simulink model "Main"  (R2022a)
settings: Solver=VariableStepAuto  StartTime=0.0  StopTime=30  RelTol=1e-3
values from neighbouring files (symbols this model uses):
  A_eq = double(A_eq)    [source_export.m]
  b = 7.66e-5    (= 7.66e-05)    [source_export.m]
  B_eq = double(B_eq)    [source_export.m]
  C = [1 0 0 0 0 0 0 0 0 0 0 0 ... (first row only)    [source_export.m]
  C_eq = C_final([1 2 3 6], 1:12)    [source_export.m]
  C_simulink = eye(12)    [source_export.m]
  Condition_0 = transpose([0 0 0 0 0 0 0 0 0 0 0 0])    [source_export.m]
  Condition_1 = transpose([0.2 0.2 0.2 0.2 0.2 0.2 0.2 0.2 0.2 0.2 0.2 0.2])    [source_export.m]
  D = zeros(4,4)    [source_export.m]
  d = 5.63e-6    (= 5.63e-06)    [source_export.m]
  D_Simulink = zeros(12,4)    [source_export.m]
  F = [      -20,   -20,   -20,   -21,   -21,   15,   -21.5, -21.5 ... (first row only)    [source_export.m]
  g = 9.81    [source_export.m]
  inv_G0 = inv_G_0( : , [1 , 2 ,3 ,6])    [source_export.m]
  inv_G0_LQR = inv_G_0_LQR( : , [1 , 2 ,3 ,6])    [source_export.m]
  Ixx = 8.5532e-3    (= 0.0085532)    [source_export.m]
  Iyy = 8.5532e-3    (= 0.0085532)    [source_export.m]
  Izz = 1.476e-2    (= 0.01476)    [source_export.m]
  K_d_LQR = K_LQR(:,1:12)    [source_export.m]
  K_q_LQR = K_LQR(:,12+1:12+4)    [source_export.m]
  Kfeedback = place(A_eq,B_eq,Poles)    [source_export.m]
  L = place(A_eq.',C_eq.',poles_obsv).'    [source_export.m]
  l = 0.22    [source_export.m]
  L_RO = 100*[1 2 1 14 ... (first row only)    [source_export.m]
  m = 1    [source_export.m]
  Q_1 = inv_mat2(:,1:q)    [source_export.m]
  Q_2 = inv_mat2(:,q+1:n)    [source_export.m]
  T_O = lyap(-F,A_eq,-L_RO*C)    [source_export.m]
undefined symbols (not defined in the file or in its folder): Discrete, K_LQR1, Time
libraries: slpidlib x8, simulink x6, ctrlSharedLib x1, sim3dlib x1, uavsim3dlib x1
(part 2 of 2)

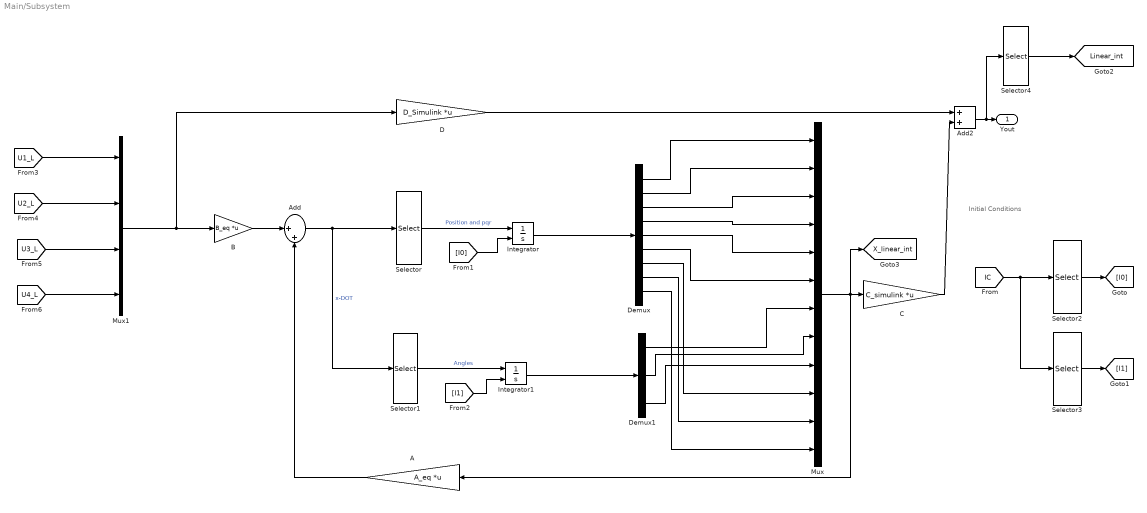
== system Main/Subsystem ==
  note: Initial Conditions
  A : Gain  Gain=A_eq  Multiplication=Matrix(K*u)
  Add : Sum  Inputs=|++
  Add2 : Sum
  B : Gain  Gain=B_eq  Multiplication=Matrix(K*u)
  C : Gain  Gain=C_simulink  Multiplication=Matrix(K*u)
  D : Gain  Gain=D_Simulink  Multiplication=Matrix(K*u)
  Demux : Demux  Outputs=9
  Demux1 : Demux  Outputs=3
  Integrator : Integrator  InitialConditionSource=external
  Integrator1 : Integrator  InitialConditionSource=external  WrapState=on
  Mux : Mux  Inputs=12
  Mux1 : Mux
  Selector : Selector  InputPortWidth=12  IndexOptions=Index vector (dialog)  Indices=[1 2 3 4 5 6 10 11 12]  OutputSizes=1
  Selector1 : Selector  InputPortWidth=12  IndexOptions=Index vector (dialog)  Indices=[7 8 9]  OutputSizes=1
  Selector2 : Selector  InputPortWidth=12  IndexOptions=Index vector (dialog)  Indices=[1 2 3 4 5 6 10 11 12]  OutputSizes=1
  Selector3 : Selector  InputPortWidth=12  IndexOptions=Index vector (dialog)  Indices=[7 8 9]  OutputSizes=1
  Selector4 : Selector  InputPortWidth=12  IndexOptions=Index vector (dialog)  Indices=[1 3 5 7 8 9]  OutputSizes=1
  Yout : Outport
  tag scope: Linear_int=global, X_linear_int=global
  wires:
  B/1 -> Add/1
  A/1 -> Add/2
  Add/1 -> Selector1/1, Selector/1  "x-DOT"
  Selector/1 -> Integrator/1  "Position and pqr"
  Selector1/1 -> Integrator1/1  "Angles"
  [IC] -> Selector3/1, Selector2/1
  Selector3/1 -> [I1]
  Selector2/1 -> [I0]
  [I1] -> Integrator1/2
  [I0] -> Integrator/2
  Integrator1/1 -> Demux1/1
  Integrator/1 -> Demux/1
  Demux/1 -> Mux/1
  Demux/2 -> Mux/2
  Demux/3 -> Mux/3
  Demux/4 -> Mux/4
  Demux/5 -> Mux/5
  Demux/6 -> Mux/6
  Demux1/1 -> Mux/7
  Demux1/2 -> Mux/8
  Demux1/3 -> Mux/9
  Demux/7 -> Mux/10
  Demux/8 -> Mux/11
  Demux/9 -> Mux/12
  D/1 -> Add2/1
  C/1 -> Add2/2
  Mux1/1 -> D/1, B/1
  [U2_L] -> Mux1/2
  [U3_L] -> Mux1/3
  [U4_L] -> Mux1/4
  Add2/1 -> Selector4/1, Yout/1
  Mux/1 -> [X_linear_int], A/1, C/1
  [U1_L] -> Mux1/1
  Selector4/1 -> [Linear_int]

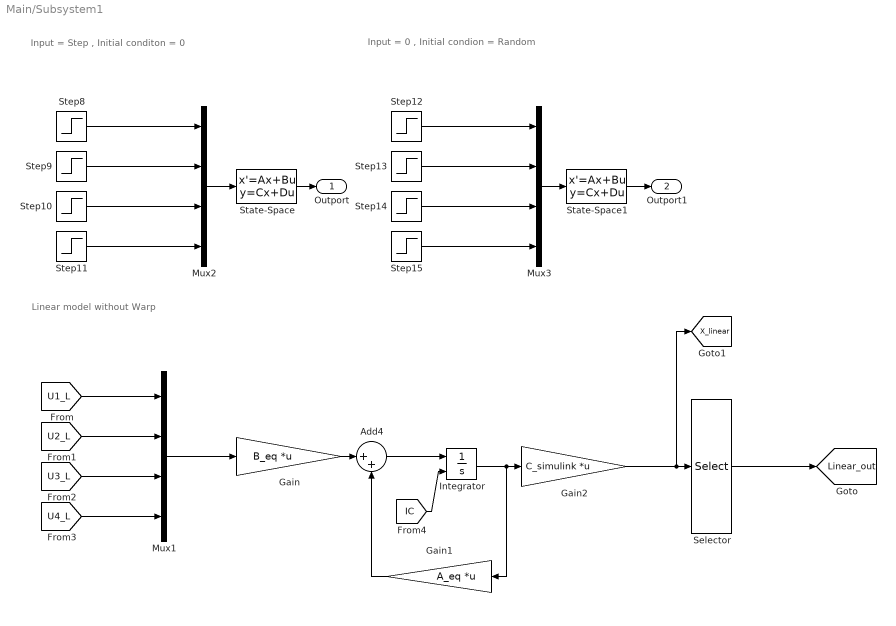
== system Main/Subsystem1 ==
  note: Linear model without Warp
  note: Input = Step , Initial conditon = 0
  note: Input = 0 , Initial condion = Random
  Add4 : Sum  Inputs=|++
  Gain : Gain  Gain=B_eq  Multiplication=Matrix(K*u)
  Gain1 : Gain  Gain=A_eq  Multiplication=Matrix(K*u)
  Gain2 : Gain  Gain=C_simulink  Multiplication=Matrix(K*u)
  Integrator : Integrator  InitialConditionSource=external
  Mux1 : Mux
  Mux2 : Mux
  Mux3 : Mux
  Selector : Selector  InputPortWidth=12  IndexOptions=Index vector (dialog)  Indices=[1 3 5 7 8 9]  OutputSizes=1
  State-Space : StateSpace  A=A_eq  B=B_eq  C=C  D=D  InitialCondition=Condition_0
  State-Space1 : StateSpace  A=A_eq  B=B_eq  C=C  D=D  InitialCondition=Condition_1
  Step{8..11} (4 alike) : Step  Time=0  SampleTime=0
  Step{12..15} (4 alike) : Step  Time=0  After=0  SampleTime=0
  Outport : Outport
  Outport1 : Outport  Port=2
  tag scope: Linear_out=global, X_linear=global
  wires:
  State-Space1/1 -> Outport1/1
  Step15/1 -> Mux3/4
  Step11/1 -> Mux2/4
  Step9/1 -> Mux2/2
  Mux3/1 -> State-Space1/1
  Step10/1 -> Mux2/3
  State-Space/1 -> Outport/1
  Step13/1 -> Mux3/2
  Mux2/1 -> State-Space/1
  Step14/1 -> Mux3/3
  [U2_L] -> Mux1/2
  [U3_L] -> Mux1/3
  [U4_L] -> Mux1/4
  Step12/1 -> Mux3/1
  [U1_L] -> Mux1/1
  Selector/1 -> [Linear_out]
  [IC] -> Integrator/2
  Integrator/1 -> Gain1/1, Gain2/1
  Gain1/1 -> Add4/2
  Mux1/1 -> Gain/1
  Gain/1 -> Add4/1
  Gain2/1 -> [X_linear], Selector/1
  Add4/1 -> Integrator/1
  Step8/1 -> Mux2/1

== system Main/Subsystem2 ==
  In1 : Inport
  Demux8 : Demux
  tag scope: i1=global, i2=global, i3=global, i4=global
  wires:
  In1/1 -> Demux8/1
  Demux8/1 -> [i1]
  Demux8/2 -> [i2]
  Demux8/3 -> [i3]
  Demux8/4 -> [i4]

== system Main/Subsystem3 ==
  Translation : Inport
  Rotation : Inport  Port=2
  Simulation 3D Scene Configuration : sim3dlib/Simulation 3D Scene Configuration  Priority=0  ProjectFormat=Default Scenes  SceneDesc=US city block  ProjectName=C:\Program Files\MATLAB\R2022b\toolbox\shared\sim3d_projects\automotive_project\UE4\WindowsNoEditor\VehicleSimulation.exe  ScenePath=/Game/Maps/USCityBlock  EnableOpenDRIVE=off  vehTagList={'Scene Origin';'SimulinkVehicle1'}  vehTag=SimulinkVehicle1  OpVisEn=off  Ts=1/60  EnableWindow=on  EnableRemoteAccess=off  EnableWeather=on  SunAltitude=90.0  SunAzimuth=147.600  clouds=26.0  wind=1  fog=14.0  rain=4.0  sensorTag=MainCamera1  sensorId=1  sensorName=MainCamera1  mountLoc=Origin  offsetFlag=off  tmountOffset=[0, 0, 0]  rmountOffset=[0, 0, 0]  HorizontalResolution=1280  VerticalResolution=720  HorizontalFOV=60  mountPoint=[0 0 0]  mountOrientation=[0 0 0]  aMode=4  ID=1  GeoTrigger=Inactive
  Simulation 3D UAV Vehicle : uavsim3dlib/Simulation 3D UAV Vehicle  Priority=-1  Mesh=Quadrotor  MeshPath=/MathWorksUAVContent/UAVs/HexaRotorUAV/HexaRotor.HexaRotor  Color=Black  ActorName=SimulinkVehicle1  InitialTranslation=[0 0 1]  InitialRotation=[0 0 0]  SampleTime=-1  ActorType=SimulinkVehicle  ID=1  aMode=4  ActorTag=SimulinkVehicle1
  wires:
  Rotation/1 -> Simulation 3D UAV Vehicle/2
  Translation/1 -> Simulation 3D UAV Vehicle/1

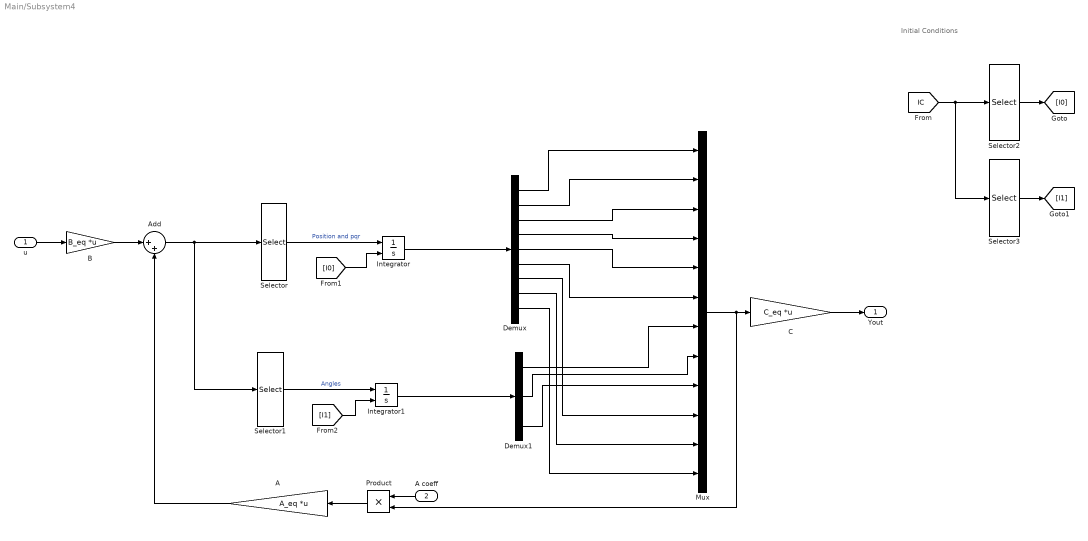
== system Main/Subsystem4 ==
  note: Initial Conditions
  u : Inport
  A coeff : Inport  Port=2
  A : Gain  Gain=A_eq  Multiplication=Matrix(K*u)
  Add : Sum  Inputs=|++
  B : Gain  Gain=B_eq  Multiplication=Matrix(K*u)
  C : Gain  Gain=C_eq  Multiplication=Matrix(K*u)
  Demux : Demux  Outputs=9
  Demux1 : Demux  Outputs=3
  Integrator : Integrator  InitialConditionSource=external
  Integrator1 : Integrator  InitialConditionSource=external  WrapState=on
  Mux : Mux  Inputs=12
  Product : Product
  Selector : Selector  InputPortWidth=12  IndexOptions=Index vector (dialog)  Indices=[1 2 3 4 5 6 10 11 12]  OutputSizes=1
  Selector1 : Selector  InputPortWidth=12  IndexOptions=Index vector (dialog)  Indices=[7 8 9]  OutputSizes=1
  Selector2 : Selector  InputPortWidth=12  IndexOptions=Index vector (dialog)  Indices=[1 2 3 4 5 6 10 11 12]  OutputSizes=1
  Selector3 : Selector  InputPortWidth=12  IndexOptions=Index vector (dialog)  Indices=[7 8 9]  OutputSizes=1
  Yout : Outport
  wires:
  B/1 -> Add/1
  A/1 -> Add/2
  Add/1 -> Selector1/1, Selector/1
  Selector/1 -> Integrator/1  "Position and pqr"
  Selector1/1 -> Integrator1/1  "Angles"
  [IC] -> Selector3/1, Selector2/1
  Selector3/1 -> [I1]
  Selector2/1 -> [I0]
  [I1] -> Integrator1/2
  [I0] -> Integrator/2
  Integrator1/1 -> Demux1/1
  Integrator/1 -> Demux/1
  Demux/1 -> Mux/1
  Demux/2 -> Mux/2
  Demux/3 -> Mux/3
  Demux/4 -> Mux/4
  Demux/5 -> Mux/5
  Demux/6 -> Mux/6
  Demux1/1 -> Mux/7
  Demux1/2 -> Mux/8
  Demux1/3 -> Mux/9
  Demux/7 -> Mux/10
  Demux/8 -> Mux/11
  Demux/9 -> Mux/12
  Mux/1 -> Product/2, C/1
  C/1 -> Yout/1
  u/1 -> B/1
  Product/1 -> A/1
  A coeff/1 -> Product/1

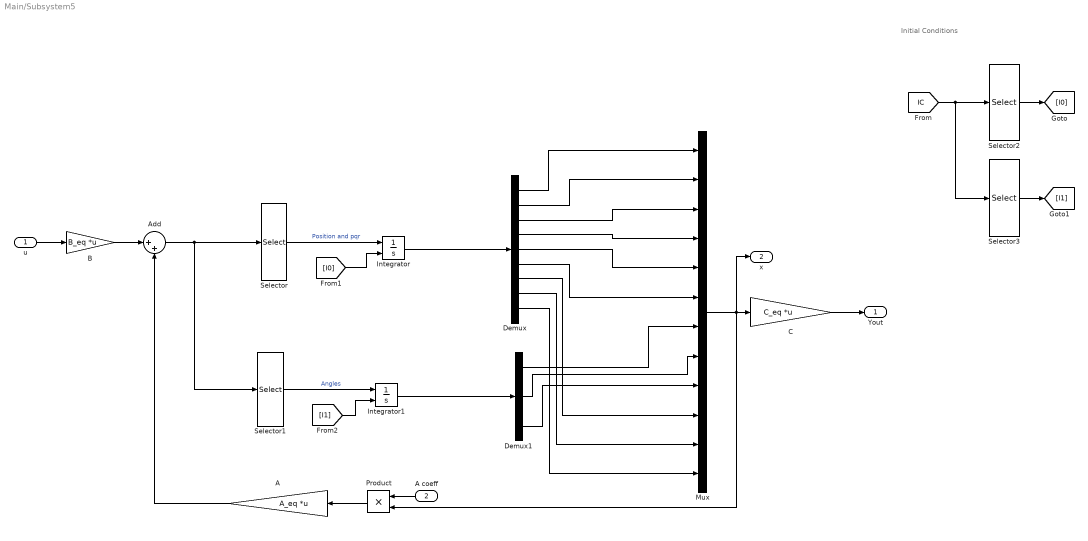
== system Main/Subsystem5 ==
  note: Initial Conditions
  u : Inport
  A coeff : Inport  Port=2
  A : Gain  Gain=A_eq  Multiplication=Matrix(K*u)
  Add : Sum  Inputs=|++
  B : Gain  Gain=B_eq  Multiplication=Matrix(K*u)
  C : Gain  Gain=C_eq  Multiplication=Matrix(K*u)
  Demux : Demux  Outputs=9
  Demux1 : Demux  Outputs=3
  Integrator : Integrator  InitialConditionSource=external
  Integrator1 : Integrator  InitialConditionSource=external  WrapState=on
  Mux : Mux  Inputs=12
  Product : Product
  Selector : Selector  InputPortWidth=12  IndexOptions=Index vector (dialog)  Indices=[1 2 3 4 5 6 10 11 12]  OutputSizes=1
  Selector1 : Selector  InputPortWidth=12  IndexOptions=Index vector (dialog)  Indices=[7 8 9]  OutputSizes=1
  Selector2 : Selector  InputPortWidth=12  IndexOptions=Index vector (dialog)  Indices=[1 2 3 4 5 6 10 11 12]  OutputSizes=1
  Selector3 : Selector  InputPortWidth=12  IndexOptions=Index vector (dialog)  Indices=[7 8 9]  OutputSizes=1
  Yout : Outport
  x : Outport  Port=2
  wires:
  B/1 -> Add/1
  A/1 -> Add/2
  Add/1 -> Selector1/1, Selector/1
  Selector/1 -> Integrator/1  "Position and pqr"
  Selector1/1 -> Integrator1/1  "Angles"
  [IC] -> Selector3/1, Selector2/1
  Selector3/1 -> [I1]
  Selector2/1 -> [I0]
  [I1] -> Integrator1/2
  [I0] -> Integrator/2
  Integrator1/1 -> Demux1/1
  Integrator/1 -> Demux/1
  Demux/1 -> Mux/1
  Demux/2 -> Mux/2
  Demux/3 -> Mux/3
  Demux/4 -> Mux/4
  Demux/5 -> Mux/5
  Demux/6 -> Mux/6
  Demux1/1 -> Mux/7
  Demux1/2 -> Mux/8
  Demux1/3 -> Mux/9
  Demux/7 -> Mux/10
  Demux/8 -> Mux/11
  Demux/9 -> Mux/12
  Mux/1 -> Product/2, x/1, C/1
  C/1 -> Yout/1
  u/1 -> B/1
  Product/1 -> A/1
  A coeff/1 -> Product/1

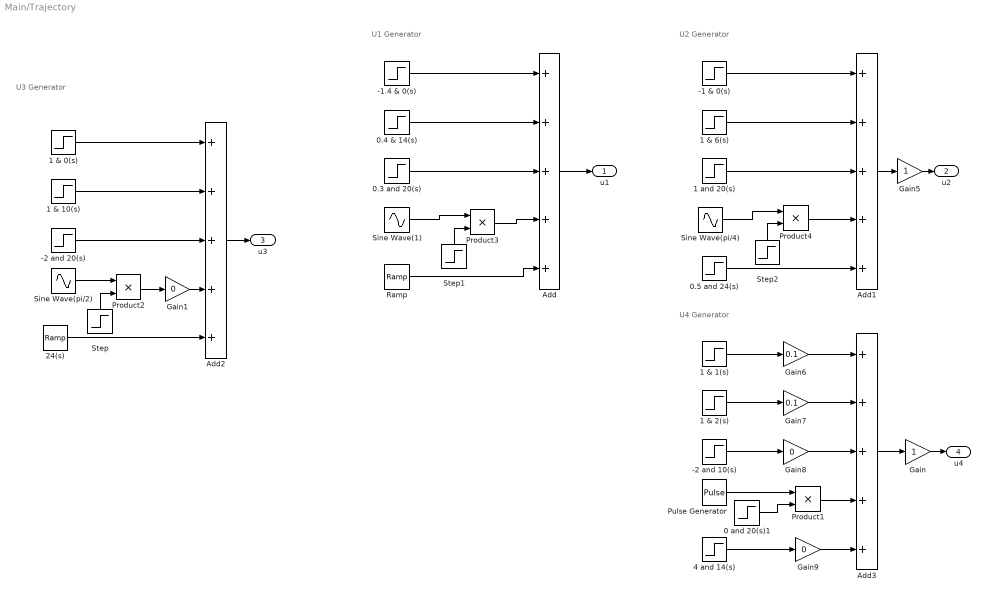
== system Main/Trajectory  ==
  note: U4 Generator
  note: U3 Generator
  note: U2 Generator
  note: U1 Generator
  -1 & 0(s) : Step  Time=0  After=-1  SampleTime=0
  -1.4 & 0(s) : Step  Time=0  After=-1.4  SampleTime=0
  -2 and 10(s) : Step  Time=10  After=-2  SampleTime=0
  -2 and 20(s) : Step  Time=20  After=-2  SampleTime=0
  0 and 20(s)1 : Step  Time=20  Before=1  After=0  SampleTime=0
  0.3 and 20(s) : Step  Time=20  After=0.3  SampleTime=0
  0.4 & 14(s) : Step  Time=14  After=0.4  SampleTime=0
  0.5 and 24(s) : Step  Time=24  After=0.5  SampleTime=0
  1 & 0(s) : Step  Time=0  After=2  SampleTime=0
  1 & 1(s) : Step  SampleTime=0
  1 & 10(s) : Step  Time=10  After=2  SampleTime=0
  1 & 2(s) : Step  Time=2  After=-1  SampleTime=0
  1 & 6(s) : Step  Time=6  SampleTime=0
  1 and 20(s) : Step  Time=20  SampleTime=0
  24(s) : simulink/Sources/Ramp  slope=1  start=24  InitialOutput=0
  4 and 14(s) : Step  Time=12  After=4  SampleTime=0
  Add{,1..3} (4 alike) : Sum  Inputs=+++++
  Gain : Gain
  Gain1 : Gain  Gain=0
  Gain5 : Gain
  Gain6 : Gain  Gain=0.1
  Gain7 : Gain  Gain=0.1
  Gain8 : Gain  Gain=0
  Gain9 : Gain  Gain=0
  Product{1..4} (4 alike) : Product
  Pulse Generator : DiscretePulseGenerator  PulseType=Time based  Period=5  PulseWidth=30  PhaseDelay=5
  Ramp : simulink/Sources/Ramp  slope=2  start=0  InitialOutput=0
  Sine Wave(1) : Sin  Amplitude=0.4  SampleTime=0
  Sine Wave(pi/2) : Sin  Amplitude=0.4  Frequency=pi/2  SampleTime=0
  Sine Wave(pi/4) : Sin  Frequency=pi/4  SampleTime=0
  Step : Step  Time=6  SampleTime=0
  Step1 : Step  Time=8  SampleTime=0
  Step2 : Step  Time=11  SampleTime=0
  u1 : Outport
  u2 : Outport  Port=2
  u3 : Outport  Port=3
  u4 : Outport  Port=4
  wires:
  Add/1 -> u1/1
  -1.4 & 0(s)/1 -> Add/1
  0.3 and 20(s)/1 -> Add/3
  0.4 & 14(s)/1 -> Add/2
  Ramp/1 -> Add/5
  0.5 and 24(s)/1 -> Add1/5
  1 & 6(s)/1 -> Add1/2
  -1 & 0(s)/1 -> Add1/1
  1 and 20(s)/1 -> Add1/3
  Add2/1 -> u3/1
  -2 and 20(s)/1 -> Add2/3
  24(s)/1 -> Add2/5
  Sine Wave(pi/2)/1 -> Product2/1
  1 & 10(s)/1 -> Add2/2
  1 & 0(s)/1 -> Add2/1
  Product2/1 -> Gain1/1
  Add3/1 -> Gain/1
  4 and 14(s)/1 -> Gain9/1
  1 & 1(s)/1 -> Gain6/1
  -2 and 10(s)/1 -> Gain8/1
  1 & 2(s)/1 -> Gain7/1
  Gain/1 -> u4/1
  Gain1/1 -> Add2/4
  Product4/1 -> Add1/4
  Add1/1 -> Gain5/1
  Gain5/1 -> u2/1
  Gain6/1 -> Add3/1
  Gain7/1 -> Add3/2
  Gain8/1 -> Add3/3
  Gain9/1 -> Add3/5
  Product1/1 -> Add3/4
  Pulse Generator/1 -> Product1/1
  0 and 20(s)1/1 -> Product1/2
  Step/1 -> Product2/2
  Sine Wave(1)/1 -> Product3/1
  Step1/1 -> Product3/2
  Product3/1 -> Add/4
  Sine Wave(pi/4)/1 -> Product4/1
  Step2/1 -> Product4/2

== system Main/pqr ==
  Integrator1 : Integrator  InitialConditionSource=external
  Integrator2 : Integrator  InitialConditionSource=external
  Integrator3 : Integrator  InitialConditionSource=external
  tag scope: p=global, q=global, r=global
  wires:
  [q0] -> Integrator2/2
  [q_dot] -> Integrator2/1
  Integrator2/1 -> [q]
  Integrator1/1 -> [p]
  [p_dot] -> Integrator1/1
  [p0] -> Integrator1/2
  [r_dot] -> Integrator3/1
  [r0] -> Integrator3/2
  Integrator3/1 -> [r]

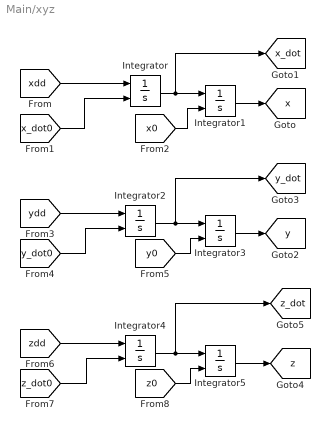
== system Main/xyz ==
  Integrator{,1..5} (6 alike) : Integrator  InitialConditionSource=external
  tag scope: x=global, x_dot=global, y=global, y_dot=global, z=global, z_dot=global
  wires:
  Integrator3/1 -> [y]
  [z0] -> Integrator5/2
  [x0] -> Integrator1/2
  Integrator2/1 -> [y_dot], Integrator3/1
  [y0] -> Integrator3/2
  Integrator/1 -> Integrator1/1, [x_dot]
  Integrator1/1 -> [x]
  Integrator4/1 -> [z_dot], Integrator5/1
  Integrator5/1 -> [z]
  [z_dot0] -> Integrator4/2
  [zdd] -> Integrator4/1
  [y_dot0] -> Integrator2/2
  [ydd] -> Integrator2/1
  [x_dot0] -> Integrator/2
  [xdd] -> Integrator/1

== system Main/Full order Observer/Dynamic Pre-compensator Observer ==
  x_hat_L : Inport
  y : Inport  Port=2
  u : Inport  Port=3
  Add : Sum  Inputs=+-
  Add3 : Sum  Inputs=--
  Integrator1 : Integrator
  Matrix Multiply1 : Product  Multiplication=Matrix(*)
  Matrix Multiply3 : Product  Multiplication=Matrix(*)
  Linear Sys input : Outport
  wires:
  u/1 -> Add/1
  y/1 -> Add/2
  Add/1 -> Integrator1/1
  Integrator1/1 -> Matrix Multiply1/2
  [Gain_Dynamic] -> Matrix Multiply1/1
  [Gain_Dyn_State] -> Matrix Multiply3/1
  x_hat_L/1 -> Matrix Multiply3/2
  Matrix Multiply1/1 -> Add3/1
  Matrix Multiply3/1 -> Add3/2
  Add3/1 -> Linear Sys input/1

== system Main/Full order Observer/Full Order Observer  ==
  y_L : Inport
  u_L - kx : Inport  Port=2
  Add2 : Sum  Inputs=+-
  Add3 : Sum  Inputs=+++
  Constant4 : Constant  Value=C_eq
  Constant5 : Constant  Value=A_eq
  Constant6 : Constant  Value=L
  Constant7 : Constant  Value=B_eq
  Integrator1 : Integrator  InitialConditionSource=external
  MatrixMultiply{4..7} (4 alike) : Product  Multiplication=Matrix(*)
  Scope : Scope
  x_hat_L : Outport
  wires:
  MatrixMultiply6/1 -> Add3/1, Scope/1  "L(y-Cx_hat)"
  Constant6/1 -> MatrixMultiply6/1
  MatrixMultiply4/1 -> Add2/2
  y_L/1 -> Add2/1
  Constant5/1 -> MatrixMultiply5/1
  Add2/1 -> MatrixMultiply6/2  "y - Cx_hat"
  u_L - kx/1 -> MatrixMultiply7/2
  Add3/1 -> Integrator1/1  "x_hat_dot"
  MatrixMultiply7/1 -> Add3/3  "Bu"
  MatrixMultiply5/1 -> Add3/2  "Ax_hat"
  Constant7/1 -> MatrixMultiply7/1
  Integrator1/1 -> x_hat_L/1, MatrixMultiply5/2, MatrixMultiply4/2
  Constant4/1 -> MatrixMultiply4/1

== system Main/Full order Observer/Full Order Observer Dynamic ==
  u_L - kx : Inport
  y_L : Inport  Port=2
  Add2 : Sum  Inputs=+-
  Add3 : Sum  Inputs=+++
  Constant4 : Constant  Value=C_eq
  Constant5 : Constant  Value=A_eq
  Constant6 : Constant  Value=L
  Constant7 : Constant  Value=B_eq
  Integrator1 : Integrator  InitialConditionSource=external
  MatrixMultiply{4..7} (4 alike) : Product  Multiplication=Matrix(*)
  Scope : Scope
  x_hat_L : Outport
  wires:
  MatrixMultiply6/1 -> Add3/1, Scope/1  "L(y-Cx_hat)"
  Constant6/1 -> MatrixMultiply6/1
  MatrixMultiply4/1 -> Add2/2
  y_L/1 -> Add2/1
  Constant5/1 -> MatrixMultiply5/1
  Add2/1 -> MatrixMultiply6/2  "y - Cx_hat"
  u_L - kx/1 -> MatrixMultiply7/2
  Add3/1 -> Integrator1/1  "x_hat_dot"
  MatrixMultiply7/1 -> Add3/3  "Bu"
  MatrixMultiply5/1 -> Add3/2  "Ax_hat"
  Constant7/1 -> MatrixMultiply7/1
  Integrator1/1 -> x_hat_L/1, MatrixMultiply5/2, MatrixMultiply4/2
  Constant4/1 -> MatrixMultiply4/1

== system Main/Full order Observer/Static Pre-compensator Observer ==
  x_hat_L : Inport
  u : Inport  Port=2
  Add1 : Sum  Inputs=-+
  Constant : Constant  Value=K_LQR1
  Constant12 : Constant  Value=inv_G0_LQR
  Matrix Multiply : Product  Multiplication=Matrix(*)
  Matrix Multiply3 : Product  Multiplication=Matrix(*)
  Linear Sys input : Outport
  wires:
  Matrix Multiply/1 -> Add1/1
  x_hat_L/1 -> Matrix Multiply/2
  Constant/1 -> Matrix Multiply/1
  u/1 -> Matrix Multiply3/2
  Matrix Multiply3/1 -> Add1/2
  Constant12/1 -> Matrix Multiply3/1
  Add1/1 -> Linear Sys input/1

== system Main/Reduced Order Observer/Dynamic Pre-compensator ==
  x_hat_L : Inport
  y : Inport  Port=2
  u : Inport  Port=3
  Add : Sum  Inputs=+-
  Add3 : Sum  Inputs=--
  Integrator1 : Integrator
  Matrix Multiply1 : Product  Multiplication=Matrix(*)
  Matrix Multiply3 : Product  Multiplication=Matrix(*)
  Linear Sys input : Outport
  wires:
  u/1 -> Add/1
  y/1 -> Add/2
  Add/1 -> Integrator1/1
  Integrator1/1 -> Matrix Multiply1/2
  [Gain_Dynamic] -> Matrix Multiply1/1
  [Gain_Dyn_State] -> Matrix Multiply3/1
  x_hat_L/1 -> Matrix Multiply3/2
  Matrix Multiply1/1 -> Add3/1
  Matrix Multiply3/1 -> Add3/2
  Add3/1 -> Linear Sys input/1

== system Main/Reduced Order Observer/Full Order Observer Reduced Static ==
  u_L - kx : Inport
  y_L : Inport  Port=2
  Add : Sum
  Add3 : Sum  Inputs=+++
  Constant : Constant  Value=Q_1
  Constant1 : Constant  Value=T_O
  Constant2 : Constant  Value=Q_2
  Constant5 : Constant  Value=F
  Constant6 : Constant  Value=L_RO
  Constant7 : Constant  Value=B_eq
  Integrator1 : Integrator
  MatrixMultiply{1..2,5..6} (4 alike) : Product  Multiplication=Matrix(*)
  MatrixMultiply7 : Product  Inputs=3  Multiplication=Matrix(*)
  x_hat_reduced : Outport
  wires:
  MatrixMultiply6/1 -> Add3/1  "Ly"
  Constant6/1 -> MatrixMultiply6/1
  Constant5/1 -> MatrixMultiply5/1
  Add3/1 -> Integrator1/1  "z_dot"
  MatrixMultiply7/1 -> Add3/3  "TBu"
  MatrixMultiply5/1 -> Add3/2  "Fz"
  Integrator1/1 -> MatrixMultiply5/2, MatrixMultiply2/2  "z"
  u_L - kx/1 -> MatrixMultiply7/3
  Constant7/1 -> MatrixMultiply7/2
  Constant1/1 -> MatrixMultiply7/1
  y_L/1 -> MatrixMultiply1/2, MatrixMultiply6/2
  Constant2/1 -> MatrixMultiply2/1
  MatrixMultiply1/1 -> Add/1  "Ly"
  MatrixMultiply2/1 -> Add/2  "Ly"
  Constant/1 -> MatrixMultiply1/1
  Add/1 -> x_hat_reduced/1

== system Main/Reduced Order Observer/Full Order Observer Reduced Static1 ==
  y_L : Inport
  u_L - kx : Inport  Port=2
  Add : Sum
  Add3 : Sum  Inputs=+++
  Constant : Constant  Value=Q_1
  Constant1 : Constant  Value=T_O
  Constant2 : Constant  Value=Q_2
  Constant5 : Constant  Value=F
  Constant6 : Constant  Value=L_RO
  Constant7 : Constant  Value=B_eq
  Integrator1 : Integrator
  MatrixMultiply{1..2,5..6} (4 alike) : Product  Multiplication=Matrix(*)
  MatrixMultiply7 : Product  Inputs=3  Multiplication=Matrix(*)
  x_hat_reduced : Outport
  wires:
  MatrixMultiply6/1 -> Add3/1  "Ly"
  Constant6/1 -> MatrixMultiply6/1
  Constant5/1 -> MatrixMultiply5/1
  Add3/1 -> Integrator1/1  "z_dot"
  MatrixMultiply7/1 -> Add3/3  "TBu"
  MatrixMultiply5/1 -> Add3/2  "Fz"
  Integrator1/1 -> MatrixMultiply5/2, MatrixMultiply2/2  "z"
  u_L - kx/1 -> MatrixMultiply7/3
  Constant7/1 -> MatrixMultiply7/2
  Constant1/1 -> MatrixMultiply7/1
  y_L/1 -> MatrixMultiply1/2, MatrixMultiply6/2
  Constant2/1 -> MatrixMultiply2/1
  MatrixMultiply1/1 -> Add/1  "Ly"
  MatrixMultiply2/1 -> Add/2  "Ly"
  Constant/1 -> MatrixMultiply1/1
  Add/1 -> x_hat_reduced/1

== system Main/Reduced Order Observer/Static Pre-compensator Reduced Observer ==
  x_hat_L : Inport
  u : Inport  Port=2
  Add1 : Sum  Inputs=-+
  Constant : Constant  Value=K_LQR1
  Constant12 : Constant  Value=inv_G0_LQR
  Matrix Multiply : Product  Multiplication=Matrix(*)
  Matrix Multiply3 : Product  Multiplication=Matrix(*)
  Linear Sys input : Outport
  wires:
  Matrix Multiply/1 -> Add1/1
  x_hat_L/1 -> Matrix Multiply/2
  Constant/1 -> Matrix Multiply/1
  u/1 -> Matrix Multiply3/2
  Matrix Multiply3/1 -> Add1/2
  Constant12/1 -> Matrix Multiply3/1
  Add1/1 -> Linear Sys input/1
